simulink subsystem "Axial_Drag"  (R2024b)
settings: Solver=VariableStepAuto  StartTime=0.0  StopTime=10.0  RelTol=1e-3
undefined symbols (not defined in the file or in its folder): Ar, CD_data, CD_input
settings Model: Creator=joedo  LastModifiedBy=finnb

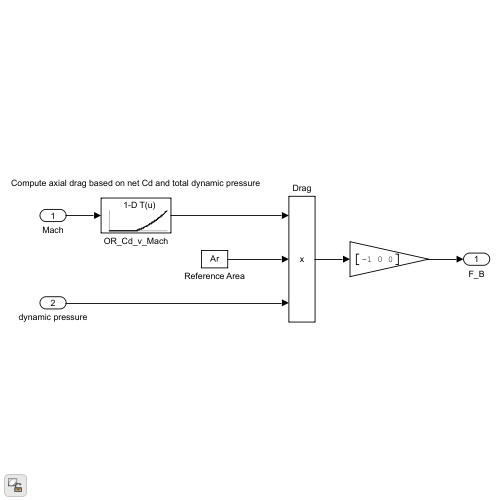
[thumbnail: Simulink's stored preview of the top-level diagram]
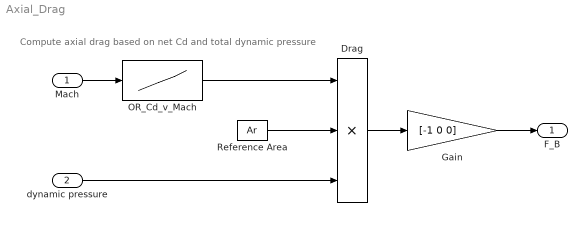
== system Axial_Drag ==
  note: Compute axial drag based on net Cd and total dynamic pressure
  Mach : Inport
  dynamic pressure : Inport  Port=2
  Drag : Product  Inputs=3
  Gain : Gain  Gain=[-1 0 0]
  OR_Cd_v_Mach : Lookup_n-D  NumberOfTableDimensions=1  BreakpointsForDimension1=CD_input  Table=CD_data  InternalRulePriority=Speed  RndMeth=Simplest
  Reference Area : Constant  Value=Ar
  F_B : Outport  VectorParamsAs1DForOutWhenUnconnected=off
  wires:
  Mach/1 -> OR_Cd_v_Mach/1
  Gain/1 -> F_B/1
  Drag/1 -> Gain/1
  OR_Cd_v_Mach/1 -> Drag/1
  dynamic pressure/1 -> Drag/3
  Reference Area/1 -> Drag/2
